simulink model "dk"  (R2022b)
settings: Solver=VariableStepAuto  StartTime=0.0  StopTime=10.0  RelTol=1e-3
undefined symbols (not defined in the file): sigbuilder_block
settings Model: Creator=Sara Rezaei  LastModifiedBy=Sara Rezaei
settings DebuggingCC: UnderSpecifiedDimensionMsg=warning

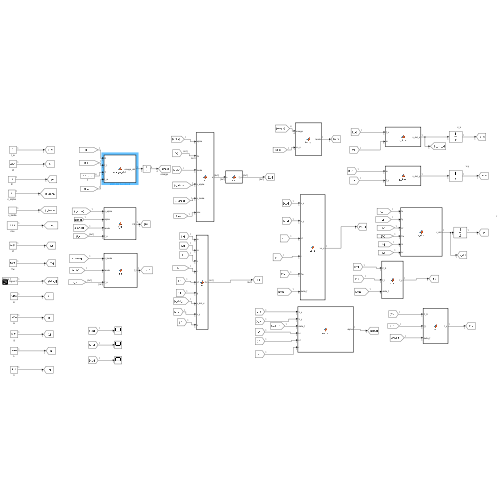
[thumbnail: Simulink's stored preview of the top-level diagram]
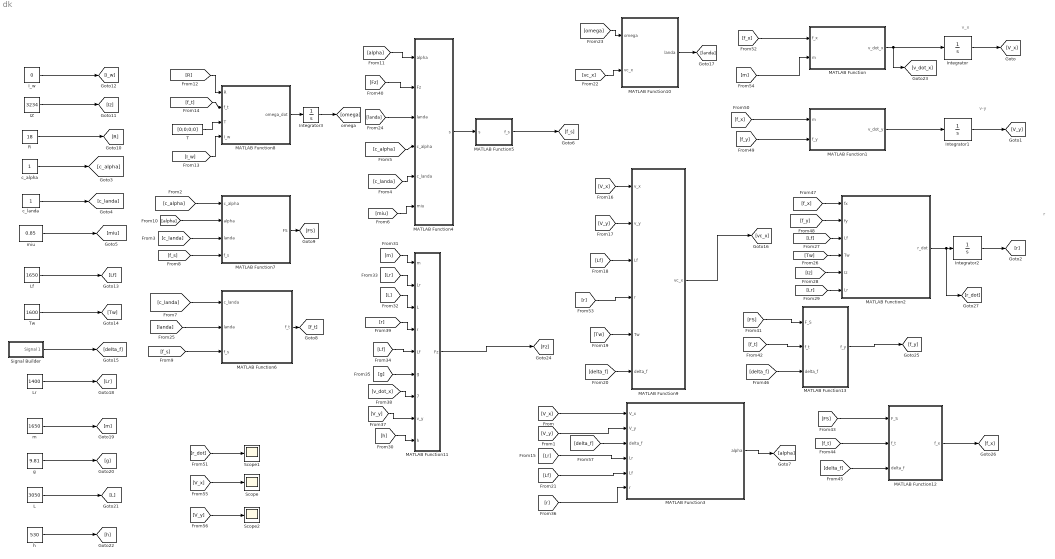
== system dk ==
  note: r
  note: v-y
  note: v_x
  IZ : Constant  Value=3234
  I_w : Constant  Value=0
  Integrator : Integrator  InitialCondition=70
  Integrator1 : Integrator
  Integrator2 : Integrator  InitialCondition=10
  Integrator3 : Integrator  InitialCondition=[0;0;0;0]
  L : Constant  Value=3050
  Lf : Constant  Value=1650
  Lr : Constant  Value=1400
  MATLAB Function : MATLAB Function  TreatAsAtomicUnit=on
  MATLAB Function1 : MATLAB Function  TreatAsAtomicUnit=on
  MATLAB Function10 : MATLAB Function  TreatAsAtomicUnit=on
  MATLAB Function11 : MATLAB Function  TreatAsAtomicUnit=on
  MATLAB Function12 : MATLAB Function  TreatAsAtomicUnit=on
  MATLAB Function13 : MATLAB Function  TreatAsAtomicUnit=on
  MATLAB Function2 : MATLAB Function  TreatAsAtomicUnit=on
  MATLAB Function3 : MATLAB Function  TreatAsAtomicUnit=on
  MATLAB Function4 : MATLAB Function  TreatAsAtomicUnit=on
  MATLAB Function5 : MATLAB Function  TreatAsAtomicUnit=on
  MATLAB Function6 : MATLAB Function  TreatAsAtomicUnit=on
  MATLAB Function7 : MATLAB Function  TreatAsAtomicUnit=on
  MATLAB Function8 : MATLAB Function  TreatAsAtomicUnit=on
  MATLAB Function9 : MATLAB Function  TreatAsAtomicUnit=on
  R : Constant  Value=18
  Scope : Scope
  Scope1 : Scope
  Scope2 : Scope
  Signal Builder : Subsystem  Tag=STV Subsys  LoadFcn=sigbuilder_block('load');  StartFcn=sigbuilder_block('start');  StopFcn=sigbuilder_block('stop');  ClipboardFcn=sigbuilder_block('clipboard');  mask(Sigbuilder block){tuvar=[0:10]}
      mask help: Simulink:masks:SigbuilderBlock_MD
      mask init:
      | if ~strcmp(get_param(bdroot(gcbh),'SimulationStatus'),'stopped') tuvar = sigbuilder_block('maskInit'); end
      settings: CopyFcn=sigbuilder_block('copy');  DeleteFcn=sigbuilder_block('delete');  ModelCloseFcn=sigbuilder_block('modelClose');  PreSaveFcn=sigbuilder_block('preSave');  PauseFcn=sigbuilder_block('pause');  ContinueFcn=sigbuilder_block('continue');  NameChangeFcn=sigbuilder_block('namechange');  OpenFcn=sigbuilder_block('open',[437.6 199.2 550.4 400 ]);  CloseFcn=sigbuilder_block('close');
      mask Display: plot(0, 0, 100, 100,[2, 2, 32, 32, 2], [68, 8, 8, 68, 68],[32, 2], [38, 38], [32, 19, 2],[53, 60, 44], [32, 17, 17, 2],[16, 16, 31, 31]);txt = getActiveGroup(gcbh);text(2, 100, txt,'verticalAlignment', 'top');
  T : Constant  Value=[0;0;0;0]
  Tw : Constant  Value=1600
  c_alpha : Constant
  c_landa : Constant
  g : Constant  Value=9.81
  h : Constant  Value=530
  m : Constant  Value=1650
  miu : Constant  Value=0.85
  wires:
  MATLAB Function/1(v_dot_x) -> [v_dot_x], Integrator/1
  Integrator/1 -> [V_x]
  MATLAB Function1/1(v_dot_y) -> Integrator1/1
  Integrator1/1 -> [V_y]
  MATLAB Function2/1(r_dot) -> [r_dot], Integrator2/1
  Integrator2/1 -> [r]
  [V_y] -> MATLAB Function3/2(V_y)
  [V_x] -> MATLAB Function3/1(V_x)
  MATLAB Function4/1(s) -> MATLAB Function5/1(s)
  [c_alpha] -> MATLAB Function7/1(c_alpha)
  c_alpha/1 -> [c_alpha]
  c_landa/1 -> [c_landa]
  miu/1 -> [miu]
  [c_landa] -> MATLAB Function7/3(landa)
  [c_landa] -> MATLAB Function4/5(c_landa)
  [c_alpha] -> MATLAB Function4/4(c_alpha)
  [miu] -> MATLAB Function4/6(miu)
  [c_landa] -> MATLAB Function6/1(c_landa)
  MATLAB Function5/1(f_s) -> [f_s]
  [f_s] -> MATLAB Function7/4(f_s)
  [f_s] -> MATLAB Function6/3(f_s)
  MATLAB Function3/1(alpha) -> [alpha]
  [alpha] -> MATLAB Function7/2(alpha)
  [alpha] -> MATLAB Function4/1(alpha)
  MATLAB Function6/1(f_t) -> [f_t]
  MATLAB Function7/1(FS) -> [FS]
  R/1 -> [R]
  IZ/1 -> [Iz]
  I_w/1 -> [I_w]
  [R] -> MATLAB Function8/1(R)
  [I_w] -> MATLAB Function8/4(I_w)
  [f_t] -> MATLAB Function8/2(f_t)
  MATLAB Function8/1(omega_dot) -> Integrator3/1
  Integrator3/1 -> [omega]
  T/1 -> MATLAB Function8/3(T)
  [V_x] -> MATLAB Function9/1(v_x)
  [V_y] -> MATLAB Function9/2(v_y)
  Lf/1 -> [Lf]
  [Lf] -> MATLAB Function9/3(Lf)
  Tw/1 -> [Tw]
  [Tw] -> MATLAB Function9/5(Tw)
  [delta_f] -> MATLAB Function9/6(delta_f)
  MATLAB Function9/1(vc_x) -> [vc_x]
  [vc_x] -> MATLAB Function10/2(vc_x)
  [omega] -> MATLAB Function10/1(omega)
  MATLAB Function10/1(landa) -> [landa]
  [landa] -> MATLAB Function4/3(landa)
  [landa] -> MATLAB Function6/2(landa)
  [Tw] -> MATLAB Function2/4(Tw)
  [Lf] -> MATLAB Function2/3(Lf)
  [Iz] -> MATLAB Function2/5(Iz)
  Lr/1 -> [Lr]
  [Lr] -> MATLAB Function2/6(Lr)
  m/1 -> [m]
  g/1 -> [g]
  L/1 -> [L]
  h/1 -> [h]
  [m] -> MATLAB Function11/1(m)
  [L] -> MATLAB Function11/3(L)
  [Lr] -> MATLAB Function11/2(Lr)
  [Lf] -> MATLAB Function11/5(Lf)
  [g] -> MATLAB Function11/6(g)
  [V_y] -> MATLAB Function11/8(v_y)
  [v_dot_x] -> MATLAB Function11/7(v_dot_x)
  [r] -> MATLAB Function11/4(r)
  [Fz] -> MATLAB Function4/2(Fz)
  MATLAB Function11/1(Fz) -> [Fz]
  [FS] -> MATLAB Function13/1(F_S)
  [f_t] -> MATLAB Function13/2(f_t)
  [FS] -> MATLAB Function12/1(F_S)
  [f_t] -> MATLAB Function12/2(f_t)
  [delta_f] -> MATLAB Function12/3(delta_f)
  [delta_f] -> MATLAB Function13/3(delta_f)
  MATLAB Function13/1(f_y) -> [f_y]
  MATLAB Function12/1(f_x) -> [f_x]
  [f_x] -> MATLAB Function2/1(fx)
  [f_y] -> MATLAB Function2/2(fy)
  [f_y] -> MATLAB Function1/2(f_y)
  [f_x] -> MATLAB Function1/1(m)
  [f_x] -> MATLAB Function/1(f_x)
  [r] -> MATLAB Function9/4(r)
  [h] -> MATLAB Function11/9(h)
  [Lf] -> MATLAB Function3/5(Lf)
  [Lr] -> MATLAB Function3/4(Lr)
  [r] -> MATLAB Function3/6(r)
  [m] -> MATLAB Function/2(m)
  [r_dot] -> Scope1/1
  [V_y] -> Scope2/1
  [V_x] -> Scope/1
  [delta_f] -> MATLAB Function3/3(delta_f)
  Signal Builder/1(Signal 1) -> [delta_f]

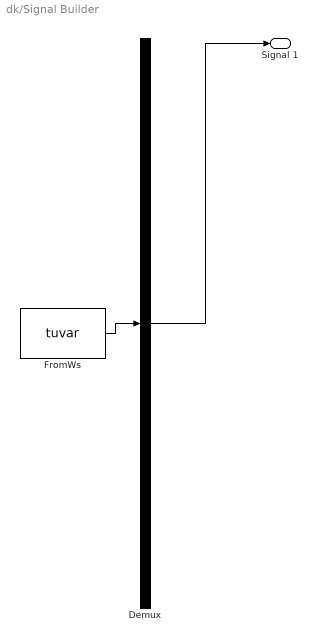
== system dk/Signal Builder ==
  Demux : Demux  Tag=STV Demux  Outputs=1
      settings: DisplayOption=none
  FromWs : FromWorkspace  Tag=STV FromWs  VariableName=tuvar
      SigBuilderData=|
      | common.afterFinalStr = 'Extrapolate'
      | common.sampleTime = 0
      | dataSet.timeRange = [0 10]
      | dataSet.name = 'Group 1'
      | sbobj.Groups.Name = 'Group 1'
      | sbobj.Groups.Signals.Name = 'Signal 1'
      | sbobj.Groups.Signals.XData = [0 4 4 6 6 10]
      | sbobj.Groups.Signals.YData = [0.455 0.455 0.995 0.99 0 0]
  Signal 1 : Outport  Tag=STV Outport
  wires:
  Demux/1 -> Signal 1/1
  FromWs/1 -> Demux/1

== matlab function dk/MATLAB Function9 ==
  data: v_x input; vc_x output; v_y input; Lf input; r input; Tw input; delta_f input
function vc_x= vc_x(v_x,v_y,Lf,r,Tw,delta_f)

vc_x = zeros(4,1);
vc_x(1)=((v_x-((r*Tw)/2))*cos(delta_f))+((v_y)+r*Lf)*sin(delta_f);
vc_x(2)=((v_x-((r*Tw)/2))*cos(delta_f))+((v_y)+r*Lf)*sin(delta_f);
vc_x(3)=v_x-(r*Tw)/2;
vc_x(4)=v_x-(r*Tw)/2;

end

== matlab function dk/MATLAB Function10 ==
  data: omega input; landa output; vc_x input
function landa = landa(omega,vc_x)

landa=zeros(4,1);
landa=(omega-vc_x)/vc_x;

end

== matlab function dk/MATLAB Function11 ==
  data: m input; Fz output; Lr input; L input; r input; Lf input; g input; v_dot_x input; v_y input; h input
function Fz= Fz(m,Lr,L,r,Lf,g,v_dot_x,v_y,h)

Fz = zeros(4,1);


        Fz(1)=((m*g)/2)*((Lr/L)-(v_dot_x-((v_y*r)/g*L)*h));

        Fz(2)=((m*g)/2)*((Lr/L)-(v_dot_x-((v_y*r)/g*L)*h));

        Fz(3)=((m*g)/2)*((Lf/L)-(v_dot_x-((v_y*r)/g*L)*h));
        
        Fz(3)=((m*g)/2)*((Lf/L)-(v_dot_x-((v_y*r)/g*L)*h));





end

== matlab function dk/MATLAB Function12 ==
  data: F_S input; f_x output; f_t input; delta_f input
function f_x = fx(F_S,f_t,delta_f)
f_x=zeros(4,1);
%delta_r=0
f_x(1)=f_t*cos(delta_f)-F_S*sin(delta_f);
f_x(2)=f_t*cos(delta_f)-F_S*sin(delta_f);
f_x(3)=f_t;
f_x(4)=f_t;

end

== matlab function dk/MATLAB Function13 ==
  data: F_S input; f_y output; f_t input; delta_f input
function f_y = f_y(F_S,f_t,delta_f)
f_y=zeros(4,1);
%delta_r=0
f_y(1)=f_t*sin(delta_f)-F_S*cos(delta_f);
f_y(2)=f_t*sin(delta_f)-F_S*cos(delta_f);
f_y(3)=F_S;
f_y(4)=F_S;


end

== matlab function dk/MATLAB Function1 ==
  data: m input; v_dot_y output; f_y input
function v_dot_y = y_2dot(m,f_y)
v_dot_y=(f_y(1)+f_y(2)+f_y(3)+f_y(4))/m;

end

== matlab function dk/MATLAB Function ==
  data: f_x input; v_dot_x output; m input
function v_dot_x = x_2dot(f_x,m)
v_dot_x=(f_x(1)+f_x(2)+f_x(3)+f_x(4))/m;




end

== matlab function dk/MATLAB Function2 ==
  data: fx input; r_dot output; fy input; Lf input; Tw input; Iz input; Lr input
function r_dot = r_dot(fx,fy,Lf,Tw,Iz,Lr)
r_dot = (Lf*(fy(1)+fy(2))-Lr(fy(3)+fy(4))+(fx(1)+fx(3)-fx(2)-fx(4))*(Tw/2))/Iz;
end

== matlab function dk/MATLAB Function3 ==
  data: V_x input; alpha output; V_y input; delta_f input; Lr input; Lf input; r input
function alpha = alpha(V_x,V_y,delta_f,Lr,Lf,r)

 alpha = zeros(4,1);

alpha(1) = delta_f - atan((Lf*r+V_y)/V_x);

alpha(2) = delta_f - atan((Lf*r+V_y)/V_x);

alpha(3) = -1*atan((Lr*r+V_y)/V_x);

alpha(4) = -1*atan((Lr*r+V_y)/V_x);

end

== matlab function dk/MATLAB Function4 ==
  data: alpha input; s output; Fz input; landa input; c_alpha input; c_landa input; miu input
function s= S(alpha,Fz,landa,c_alpha,c_landa,miu)

s= zeros(4,1);

for i=1:4

    s = (miu*Fz(i)*(1+landa))/(2*(sqrt((c_landa*landa)^2+(c_alpha*tan(alpha)^2))));


end

== matlab function dk/MATLAB Function5 ==
  data: s input; f_s output
function f_s = f_s(s)
 f_s=zeros(4,1);
for i=1:1:4
    if s(i)<1
    f_s=(2-s(i))*s(i);
else 
    f_s=1;
end



end

== matlab function dk/MATLAB Function6 ==
  data: c_landa input; f_t output; landa input; f_s input
function f_t = f_t(c_landa,landa,f_s)
f_t=zeros(4,1);

f_t=(c_landa*landa*f_s)/(1+landa);

end

== matlab function dk/MATLAB Function7 ==
  data: c_alpha input; FS output; alpha input; landa input; f_s input
function FS= F_S(c_alpha,alpha,landa,f_s)
FS=zeros(4,1);
FS=(c_alpha*alpha)*f_s/(1+landa);
end

== matlab function dk/MATLAB Function8 ==
  data: R input; omega_dot output; f_t input; T input; I_w input
function omega_dot= omega_dot(R,f_t,T,I_w) 

omega_dot= zeros(4,1);
omega_dot=(T-(f_t*R))/I_w;

end
